simulink library "halin"  (R2021b)
settings: Solver=VariableStepAuto  StartTime=0.0  StopTime=10.0  RelTol=1e-3
undefined symbols (not defined in the file): KHAL_CAN1ABM1E2E_flg, KHAL_CAN1ESC1E2E_flg, KHAL_CAN1ESC5E2E_flg, KHAL_CAN1ESC7E2E_flg, KHAL_CAN1FCM2E2E_flg, KHAL_CAN1FCM3E2E_flg, KHAL_CAN1FCM4E2E_flg, KHAL_CAN3BMS1E2E_flg, KHAL_CAN3BMS6E2E_flg, KHAL_CAN3CCU1E2E_flg, KHAL_CAN3CCU2E2E_flg, KHAL_CAN3MCUF1E2E_flg, KHAL_CAN3MCUR1E2E_flg, KHAL_CAN3Shifter1E2E_flg, TRUE
libraries: simulink x420, FVT_lib x149, hcu_lib x49
(part 9 of 14)

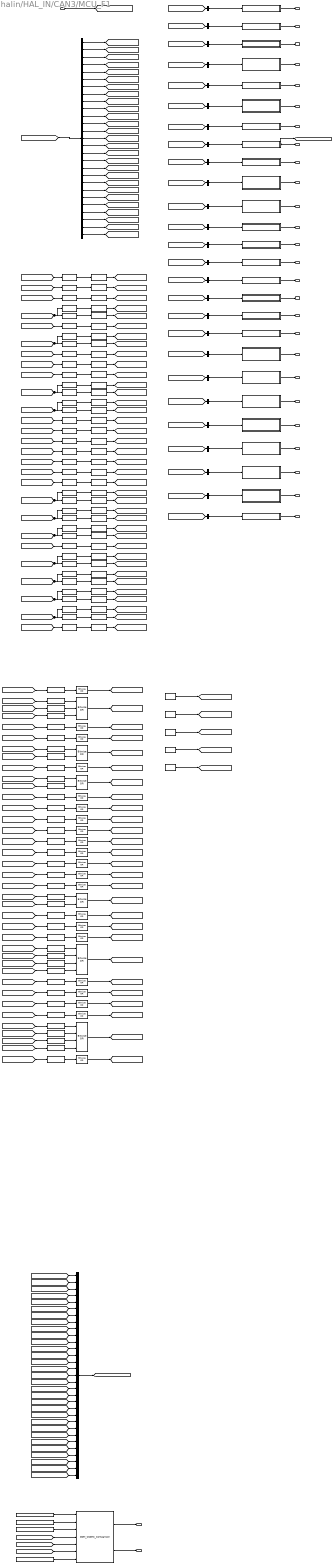
== system halin/HAL_IN/CAN3/MCU_F1 ==
  DT_CAN3_SG_MCU_F1 : Inport
  0x95 : Constant  Value=0x95
  0xf9 : Constant  Value=0xf9
  BitwiseAND{,1..37} (38 alike) : simulink/Logic and Bit Operations/Bitwise Operator  logicop=AND  UseBitMask=on  BitMask=0xFF  BitMaskRealWorld=Stored Integer
  BitwiseOR{,2..3,5,7..15,17..19,21..24,26} (21 alike) : simulink/Logic and Bit Operations/Bitwise Operator  logicop=OR  UseBitMask=off  BitMask=bin2dec('11011001')  BitMaskRealWorld=Stored Integer
  BitwiseOR1 : simulink/Logic and Bit Operations/Bitwise Operator  logicop=OR  UseBitMask=off  NumInputPorts=3  BitMask=bin2dec('11011001')  BitMaskRealWorld=Stored Integer
  BitwiseOR16 : simulink/Logic and Bit Operations/Bitwise Operator  logicop=OR  UseBitMask=off  NumInputPorts=2  BitMask=bin2dec('11011001')  BitMaskRealWorld=Stored Integer
  BitwiseOR20 : simulink/Logic and Bit Operations/Bitwise Operator  logicop=OR  UseBitMask=off  NumInputPorts=4  BitMask=bin2dec('11011001')  BitMaskRealWorld=Stored Integer
  BitwiseOR25 : simulink/Logic and Bit Operations/Bitwise Operator  logicop=OR  UseBitMask=off  NumInputPorts=4  BitMask=bin2dec('11011001')  BitMaskRealWorld=Stored Integer
  BitwiseOR4 : simulink/Logic and Bit Operations/Bitwise Operator  logicop=OR  UseBitMask=off  NumInputPorts=2  BitMask=bin2dec('11011001')  BitMaskRealWorld=Stored Integer
  BitwiseOR6 : simulink/Logic and Bit Operations/Bitwise Operator  logicop=OR  UseBitMask=off  NumInputPorts=2  BitMask=bin2dec('11011001')  BitMaskRealWorld=Stored Integer
  DDM_CS&RC_Comparison : FVT_lib/hal/DDM_CS&RC_Comparison  MsgCycleTime=10
  Data Type Conversion{,1..37} (38 alike) : DataTypeConversion  OutDataTypeStr=uint8
  FrActvDmpDisabSta : Subsystem
  FrEDUDrtSta : Subsystem
  FrEDUOpratingSta : Subsystem
  FrEDURealTMTq : Subsystem
  FrEDURotateDirction : Subsystem
  FrEDUTqReqFbk : Subsystem
  FrMCU1Chksum : Subsystem
  FrMCU1RolCnt : Subsystem
  FrMCUBAT : Subsystem
  FrMCUDCBusCurr : Subsystem
  FrMCUDCBusVolt : Subsystem
  FrMCUDischrgSta : Subsystem
  FrMCUEnaSta : Subsystem
  FrMCUErr : Subsystem
  FrMCUIGNsta : Subsystem
  FrMCUReady : Subsystem
  FrMCUReady4Pre : Subsystem
  FrMCUSysSta : Subsystem
  FrMCUTemp : Subsystem
  FrMotorAvailTq : Subsystem
  FrRegenAvailTq : Subsystem
  FrTMSpd : Subsystem
  FrTMTemp : Subsystem
  FrTMid : Subsystem
  FrTMiq : Subsystem
  KHAL_CAN3MCUF1E2E_flg : Constant  Value=KHAL_CAN3MCUF1E2E_flg
  LeftShift : ArithShift  BitShiftNumber=1  BitShiftDirection=Left
  LeftShift1 : ArithShift  BitShiftNumber=2  BitShiftDirection=Left
  LeftShift{4,6,9..10,12..13,15} (7 alike) : ArithShift  BitShiftDirection=Left
  LeftShift11 : ArithShift  BitShiftNumber=3  BitShiftDirection=Left
  LeftShift14 : ArithShift  BitShiftNumber=1  BitShiftDirection=Left
  LeftShift2 : ArithShift  BitShiftNumber=5  BitShiftDirection=Left
  LeftShift3 : ArithShift  BitShiftNumber=6  BitShiftDirection=Left
  LeftShift5 : ArithShift  BitShiftNumber=4  BitShiftDirection=Left
  LeftShift7 : ArithShift  BitShiftNumber=3  BitShiftDirection=Left
  LeftShift8 : ArithShift  BitShiftNumber=4  BitShiftDirection=Left
  MCUWarnF : Subsystem
  MessageRollingCounter : FVT_lib/hal/MessageRollingCounter  CounterMAX=14  task_time_ms=5  msg_time_ms=10
  Mux : Mux  Inputs=31
  RightShift{,2,4,6,10,14,16,18,20} (9 alike) : ArithShift  BitShiftNumber=8
  RightShift{1,3,5,7,11,15,17,19,21} (9 alike) : ArithShift
  RightShift12 : ArithShift  BitShiftNumber=4
  RightShift13 : ArithShift  BitShiftNumber=-4
  RightShift8 : ArithShift  BitShiftNumber=1
  RightShift9 : ArithShift  BitShiftNumber=-7
  bus_selector : BusSelector  OutputSignals=CAN3_Fr_ActvDmpDisabSta,CAN3_Fr_EDUDrtSta,CAN3_Fr_EDUOpratingSta,CAN3_Fr_EDURealTMTq,CAN3_Fr_EDURotateDirction,CAN3_Fr_EDUTqReqFbk,CAN3_Fr_MCU1Chksum,CAN3_Fr_MCU1RolCnt,CAN3_Fr_MCUBAT,CAN3_Fr_MCUDCBusCurr,CAN3_Fr_MCUDCBusVolt,CAN3_Fr_MCUDischrgSta,CAN3_Fr_MCUEnaSta,CAN3_Fr_MCUErr,CAN3_Fr_MCUIGN_sta,CAN3_Fr_MCUReady,CAN3_Fr_MCUReady4Pre,CAN3_Fr_MCUSysSta,CAN3_Fr_MCUTemp,CAN3_Fr_MotorAvailTq,CAN3_Fr_RegenAvailTq,CAN3_Fr_Reserved_bits,CAN3_Fr_TMSpd,CAN3_Fr_TMTemp,CAN3_Fr_TMid,CAN3_Fr_TMiq,CAN3_MCUWarn_F
  bus_selector1 : BusSelector  OutputSignals=CAN3_Fr_ActvDmpDisabSta
  bus_selector10 : BusSelector  OutputSignals=CAN3_Fr_MCUDCBusCurr
  bus_selector11 : BusSelector  OutputSignals=CAN3_Fr_MCUDCBusVolt
  bus_selector12 : BusSelector  OutputSignals=CAN3_Fr_MCUDischrgSta
  bus_selector13 : BusSelector  OutputSignals=CAN3_Fr_MCUEnaSta
  bus_selector14 : BusSelector  OutputSignals=CAN3_Fr_MCUErr
  bus_selector15 : BusSelector  OutputSignals=CAN3_Fr_MCUIGN_sta
  bus_selector16 : BusSelector  OutputSignals=CAN3_Fr_MCUReady
  bus_selector17 : BusSelector  OutputSignals=CAN3_Fr_MCUReady4Pre
  bus_selector18 : BusSelector  OutputSignals=CAN3_Fr_MCUSysSta
  bus_selector19 : BusSelector  OutputSignals=CAN3_Fr_MCUTemp
  bus_selector2 : BusSelector  OutputSignals=CAN3_Fr_EDUDrtSta
  bus_selector20 : BusSelector  OutputSignals=CAN3_Fr_MotorAvailTq
  bus_selector21 : BusSelector  OutputSignals=CAN3_Fr_RegenAvailTq
  bus_selector22 : BusSelector  OutputSignals=CAN3_Fr_TMSpd
  bus_selector23 : BusSelector  OutputSignals=CAN3_Fr_TMTemp
  bus_selector24 : BusSelector  OutputSignals=CAN3_Fr_TMid
  bus_selector25 : BusSelector  OutputSignals=CAN3_Fr_TMiq
  bus_selector26 : BusSelector  OutputSignals=CAN3_MCUWarn_F
  bus_selector3 : BusSelector  OutputSignals=CAN3_Fr_EDUOpratingSta
  bus_selector4 : BusSelector  OutputSignals=CAN3_Fr_EDURealTMTq
  bus_selector5 : BusSelector  OutputSignals=CAN3_Fr_EDURotateDirction
  bus_selector6 : BusSelector  OutputSignals=CAN3_Fr_EDUTqReqFbk
  bus_selector7 : BusSelector  OutputSignals=CAN3_Fr_MCU1Chksum
  bus_selector8 : BusSelector  OutputSignals=CAN3_Fr_MCU1RolCnt
  bus_selector9 : BusSelector  OutputSignals=CAN3_Fr_MCUBAT
  constant{,1..4} (5 alike) : Constant  Value=0x0  OutDataTypeStr=uint8
  VHAL_MCUF1CSErr_flg : Outport
  VHAL_MCUF1RCErr_flg : Outport  Port=2
  VHAL_FrActvDmpDisabSta_flg : Outport  Port=3
  VHAL_FrEDUDrtSta_flg : Outport  Port=4
  VHAL_FrEDUOpratingSta_flg : Outport  Port=5
  VHAL_FrEDURealTMTq_Nm : Outport  Port=6
  VHAL_FrEDURotateDirction_enum : Outport  Port=7
  VHAL_FrEDUTqReqFbk_Nm : Outport  Port=8
  VHAL_FrMCU1Chksum_enum : Outport  Port=9
  VHAL_FrMCU1RolCnt_enum : Outport  Port=10
  VHAL_FrMCUBAT_V : Outport  Port=11
  VHAL_FrMCUDCBusCurr_A : Outport  Port=12
  VHAL_FrMCUDCBusVolt_V : Outport  Port=13
  VHAL_FrMCUDischrgSta_flg : Outport  Port=14
  VHAL_FrMCUEnaSta_flg : Outport  Port=15
  VHAL_FrMCUErr_enum : Outport  Port=16
  VHAL_FrMCUIGNsta_flg : Outport  Port=17
  VHAL_FrMCUReady_flg : Outport  Port=18
  VHAL_FrMCUReady4Pre_flg : Outport  Port=19
  VHAL_FrMCUSysSta_enum : Outport  Port=20
  VHAL_FrMCUTemp_C : Outport  Port=21
  VHAL_FrMotorAvailTq_Nm : Outport  Port=22
  VHAL_FrRegenAvailTq_Nm : Outport  Port=23
  VHAL_FrTMSpd_rpm : Outport  Port=24
  VHAL_FrTMTemp_C : Outport  Port=25
  VHAL_FrTMid_A : Outport  Port=26
  VHAL_FrTMiq_A : Outport  Port=27
  VHAL_MCUWarnF_enum : Outport  Port=28
  wires:
  DT_CAN3_SG_MCU_F1/1 -> [DT_CAN3_SG_MCU_F1]
  [DT_CAN3_SG_MCU_F1] -> bus_selector/1
  bus_selector/1 -> [CAN3_Fr_ActvDmpDisabSta]  "<CAN3_Fr_ActvDmpDisabSta>"
  [CAN3_Fr_ActvDmpDisabSta] -> LeftShift/1
  LeftShift/1 -> BitwiseAND/1
  BitwiseAND/1 -> [Byte_25_CAN3_Fr_ActvDmpDisabSta]
  bus_selector/2 -> [CAN3_Fr_EDUDrtSta]  "<CAN3_Fr_EDUDrtSta>"
  [CAN3_Fr_EDUDrtSta] -> LeftShift1/1
  LeftShift1/1 -> BitwiseAND1/1
  BitwiseAND1/1 -> [Byte_25_CAN3_Fr_EDUDrtSta]
  bus_selector/3 -> [CAN3_Fr_EDUOpratingSta]  "<CAN3_Fr_EDUOpratingSta>"
  [CAN3_Fr_EDUOpratingSta] -> LeftShift2/1
  LeftShift2/1 -> BitwiseAND2/1
  BitwiseAND2/1 -> [Byte_30_CAN3_Fr_EDUOpratingSta]
  bus_selector/4 -> [CAN3_Fr_EDURealTMTq]  "<CAN3_Fr_EDURealTMTq>"
  [CAN3_Fr_EDURealTMTq] -> RightShift/1, RightShift1/1
  RightShift/1 -> BitwiseAND3/1
  BitwiseAND3/1 -> [Byte_28_CAN3_Fr_EDURealTMTq]
  RightShift1/1 -> BitwiseAND4/1
  BitwiseAND4/1 -> [Byte_29_CAN3_Fr_EDURealTMTq]
  bus_selector/5 -> [CAN3_Fr_EDURotateDirction]  "<CAN3_Fr_EDURotateDirction>"
  [CAN3_Fr_EDURotateDirction] -> LeftShift3/1
  LeftShift3/1 -> BitwiseAND5/1
  BitwiseAND5/1 -> [Byte_30_CAN3_Fr_EDURotateDirction]
  bus_selector/6 -> [CAN3_Fr_EDUTqReqFbk]  "<CAN3_Fr_EDUTqReqFbk>"
  [CAN3_Fr_EDUTqReqFbk] -> RightShift2/1, RightShift3/1
  RightShift2/1 -> BitwiseAND6/1
  BitwiseAND6/1 -> [Byte_30_CAN3_Fr_EDUTqReqFbk]
  RightShift3/1 -> BitwiseAND7/1
  BitwiseAND7/1 -> [Byte_31_CAN3_Fr_EDUTqReqFbk]
  bus_selector/7 -> [CAN3_Fr_MCU1Chksum]  "<CAN3_Fr_MCU1Chksum>"
  [CAN3_Fr_MCU1Chksum] -> LeftShift4/1
  LeftShift4/1 -> BitwiseAND8/1
  BitwiseAND8/1 -> [Byte_0_CAN3_Fr_MCU1Chksum]
  bus_selector/8 -> [CAN3_Fr_MCU1RolCnt]  "<CAN3_Fr_MCU1RolCnt>"
  [CAN3_Fr_MCU1RolCnt] -> LeftShift5/1
  LeftShift5/1 -> BitwiseAND9/1
  BitwiseAND9/1 -> [Byte_1_CAN3_Fr_MCU1RolCnt]
  bus_selector/9 -> [CAN3_Fr_MCUBAT]  "<CAN3_Fr_MCUBAT>"
  [CAN3_Fr_MCUBAT] -> LeftShift6/1
  LeftShift6/1 -> BitwiseAND10/1
  BitwiseAND10/1 -> [Byte_8_CAN3_Fr_MCUBAT]
  bus_selector/10 -> [CAN3_Fr_MCUDCBusCurr]  "<CAN3_Fr_MCUDCBusCurr>"
  [CAN3_Fr_MCUDCBusCurr] -> RightShift4/1, RightShift5/1
  RightShift4/1 -> BitwiseAND11/1
  BitwiseAND11/1 -> [Byte_21_CAN3_Fr_MCUDCBusCurr]
  RightShift5/1 -> BitwiseAND12/1
  BitwiseAND12/1 -> [Byte_22_CAN3_Fr_MCUDCBusCurr]
  bus_selector/11 -> [CAN3_Fr_MCUDCBusVolt]  "<CAN3_Fr_MCUDCBusVolt>"
  [CAN3_Fr_MCUDCBusVolt] -> RightShift6/1, RightShift7/1
  RightShift6/1 -> BitwiseAND13/1
  BitwiseAND13/1 -> [Byte_23_CAN3_Fr_MCUDCBusVolt]
  RightShift7/1 -> BitwiseAND14/1
  BitwiseAND14/1 -> [Byte_24_CAN3_Fr_MCUDCBusVolt]
  bus_selector/12 -> [CAN3_Fr_MCUDischrgSta]  "<CAN3_Fr_MCUDischrgSta>"
  [CAN3_Fr_MCUDischrgSta] -> LeftShift7/1
  LeftShift7/1 -> BitwiseAND15/1
  BitwiseAND15/1 -> [Byte_25_CAN3_Fr_MCUDischrgSta]
  bus_selector/13 -> [CAN3_Fr_MCUEnaSta]  "<CAN3_Fr_MCUEnaSta>"
  [CAN3_Fr_MCUEnaSta] -> LeftShift8/1
  LeftShift8/1 -> BitwiseAND16/1
  BitwiseAND16/1 -> [Byte_30_CAN3_Fr_MCUEnaSta]
  bus_selector/14 -> [CAN3_Fr_MCUErr]  "<CAN3_Fr_MCUErr>"
  [CAN3_Fr_MCUErr] -> LeftShift9/1
  LeftShift9/1 -> BitwiseAND17/1
  BitwiseAND17/1 -> [Byte_17_CAN3_Fr_MCUErr]
  bus_selector/15 -> [CAN3_Fr_MCUIGN_sta]  "<CAN3_Fr_MCUIGN_sta>"
  [CAN3_Fr_MCUIGN_sta] -> LeftShift10/1
  LeftShift10/1 -> BitwiseAND18/1
  BitwiseAND18/1 -> [Byte_9_CAN3_Fr_MCUIGN_sta]
  bus_selector/16 -> [CAN3_Fr_MCUReady]  "<CAN3_Fr_MCUReady>"
  [CAN3_Fr_MCUReady] -> LeftShift11/1
  LeftShift11/1 -> BitwiseAND19/1
  BitwiseAND19/1 -> [Byte_1_CAN3_Fr_MCUReady]
  bus_selector/17 -> [CAN3_Fr_MCUReady4Pre]  "<CAN3_Fr_MCUReady4Pre>"
  [CAN3_Fr_MCUReady4Pre] -> LeftShift12/1
  LeftShift12/1 -> BitwiseAND20/1
  BitwiseAND20/1 -> [Byte_25_CAN3_Fr_MCUReady4Pre]
  bus_selector/18 -> [CAN3_Fr_MCUSysSta]  "<CAN3_Fr_MCUSysSta>"
  [CAN3_Fr_MCUSysSta] -> LeftShift13/1
  LeftShift13/1 -> BitwiseAND21/1
  BitwiseAND21/1 -> [Byte_7_CAN3_Fr_MCUSysSta]
  bus_selector/19 -> [CAN3_Fr_MCUTemp]  "<CAN3_Fr_MCUTemp>"
  [CAN3_Fr_MCUTemp] -> RightShift8/1, RightShift9/1
  RightShift8/1 -> BitwiseAND22/1
  BitwiseAND22/1 -> [Byte_20_CAN3_Fr_MCUTemp]
  RightShift9/1 -> BitwiseAND23/1
  BitwiseAND23/1 -> [Byte_21_CAN3_Fr_MCUTemp]
  bus_selector/20 -> [CAN3_Fr_MotorAvailTq]  "<CAN3_Fr_MotorAvailTq>"
  [CAN3_Fr_MotorAvailTq] -> RightShift10/1, RightShift11/1
  RightShift10/1 -> BitwiseAND24/1
  BitwiseAND24/1 -> [Byte_11_CAN3_Fr_MotorAvailTq]
  RightShift11/1 -> BitwiseAND25/1
  BitwiseAND25/1 -> [Byte_12_CAN3_Fr_MotorAvailTq]
  bus_selector/21 -> [CAN3_Fr_RegenAvailTq]  "<CAN3_Fr_RegenAvailTq>"
  [CAN3_Fr_RegenAvailTq] -> RightShift12/1, RightShift13/1
  RightShift12/1 -> BitwiseAND26/1
  BitwiseAND26/1 -> [Byte_10_CAN3_Fr_RegenAvailTq]
  RightShift13/1 -> BitwiseAND27/1
  BitwiseAND27/1 -> [Byte_11_CAN3_Fr_RegenAvailTq]
  bus_selector/22 -> [CAN3_Fr_Reserved_bits]  "<CAN3_Fr_Reserved_bits>"
  [CAN3_Fr_Reserved_bits] -> LeftShift14/1
  LeftShift14/1 -> BitwiseAND28/1
  BitwiseAND28/1 -> [Byte_9_CAN3_Fr_Reserved_bits]
  bus_selector/23 -> [CAN3_Fr_TMSpd]  "<CAN3_Fr_TMSpd>"
  [CAN3_Fr_TMSpd] -> RightShift14/1, RightShift15/1
  RightShift14/1 -> BitwiseAND29/1
  BitwiseAND29/1 -> [Byte_26_CAN3_Fr_TMSpd]
  RightShift15/1 -> BitwiseAND30/1
  BitwiseAND30/1 -> [Byte_27_CAN3_Fr_TMSpd]
  bus_selector/24 -> [CAN3_Fr_TMTemp]  "<CAN3_Fr_TMTemp>"
  [CAN3_Fr_TMTemp] -> RightShift16/1, RightShift17/1
  RightShift16/1 -> BitwiseAND31/1
  BitwiseAND31/1 -> [Byte_18_CAN3_Fr_TMTemp]
  RightShift17/1 -> BitwiseAND32/1
  BitwiseAND32/1 -> [Byte_19_CAN3_Fr_TMTemp]
  bus_selector/25 -> [CAN3_Fr_TMid]  "<CAN3_Fr_TMid>"
  [CAN3_Fr_TMid] -> RightShift18/1, RightShift19/1
  RightShift18/1 -> BitwiseAND33/1
  BitwiseAND33/1 -> [Byte_15_CAN3_Fr_TMid]
  RightShift19/1 -> BitwiseAND34/1
  BitwiseAND34/1 -> [Byte_16_CAN3_Fr_TMid]
  bus_selector/26 -> [CAN3_Fr_TMiq]  "<CAN3_Fr_TMiq>"
  [CAN3_Fr_TMiq] -> RightShift20/1, RightShift21/1
  RightShift20/1 -> BitwiseAND35/1
  BitwiseAND35/1 -> [Byte_13_CAN3_Fr_TMiq]
  RightShift21/1 -> BitwiseAND36/1
  BitwiseAND36/1 -> [Byte_14_CAN3_Fr_TMiq]
  bus_selector/27 -> [CAN3_MCUWarn_F]  "<CAN3_MCUWarn_F>"
  [CAN3_MCUWarn_F] -> LeftShift15/1
  LeftShift15/1 -> BitwiseAND37/1
  BitwiseAND37/1 -> [Byte_1_CAN3_MCUWarn_F]
  Data Type Conversion/1 -> BitwiseOR/1
  [Byte_0_CAN3_Fr_MCU1Chksum] -> Data Type Conversion/1
  BitwiseOR/1 -> [Byte_0]
  Data Type Conversion1/1 -> BitwiseOR1/1
  [Byte_1_CAN3_Fr_MCU1RolCnt] -> Data Type Conversion1/1
  Data Type Conversion2/1 -> BitwiseOR1/2
  [Byte_1_CAN3_Fr_MCUReady] -> Data Type Conversion2/1
  Data Type Conversion3/1 -> BitwiseOR1/3
  [Byte_1_CAN3_MCUWarn_F] -> Data Type Conversion3/1
  BitwiseOR1/1 -> [Byte_1]
  constant/1 -> [Byte_2]
  constant1/1 -> [Byte_3]
  constant2/1 -> [Byte_4]
  constant3/1 -> [Byte_5]
  constant4/1 -> [Byte_6]
  Data Type Conversion4/1 -> BitwiseOR2/1
  [Byte_7_CAN3_Fr_MCUSysSta] -> Data Type Conversion4/1
  BitwiseOR2/1 -> [Byte_7]
  Data Type Conversion5/1 -> BitwiseOR3/1
  [Byte_8_CAN3_Fr_MCUBAT] -> Data Type Conversion5/1
  BitwiseOR3/1 -> [Byte_8]
  Data Type Conversion6/1 -> BitwiseOR4/1
  [Byte_9_CAN3_Fr_MCUIGN_sta] -> Data Type Conversion6/1
  Data Type Conversion7/1 -> BitwiseOR4/2
  [Byte_9_CAN3_Fr_Reserved_bits] -> Data Type Conversion7/1
  BitwiseOR4/1 -> [Byte_9]
  Data Type Conversion8/1 -> BitwiseOR5/1
  [Byte_10_CAN3_Fr_RegenAvailTq] -> Data Type Conversion8/1
  BitwiseOR5/1 -> [Byte_10]
  Data Type Conversion9/1 -> BitwiseOR6/1
  [Byte_11_CAN3_Fr_MotorAvailTq] -> Data Type Conversion9/1
  Data Type Conversion10/1 -> BitwiseOR6/2
  [Byte_11_CAN3_Fr_RegenAvailTq] -> Data Type Conversion10/1
  BitwiseOR6/1 -> [Byte_11]
  Data Type Conversion11/1 -> BitwiseOR7/1
  [Byte_12_CAN3_Fr_MotorAvailTq] -> Data Type Conversion11/1
  BitwiseOR7/1 -> [Byte_12]
  Data Type Conversion12/1 -> BitwiseOR8/1
  [Byte_13_CAN3_Fr_TMiq] -> Data Type Conversion12/1
  BitwiseOR8/1 -> [Byte_13]
  Data Type Conversion13/1 -> BitwiseOR9/1
  [Byte_14_CAN3_Fr_TMiq] -> Data Type Conversion13/1
  BitwiseOR9/1 -> [Byte_14]
  Data Type Conversion14/1 -> BitwiseOR10/1
  [Byte_15_CAN3_Fr_TMid] -> Data Type Conversion14/1
  BitwiseOR10/1 -> [Byte_15]
  Data Type Conversion15/1 -> BitwiseOR11/1
  [Byte_16_CAN3_Fr_TMid] -> Data Type Conversion15/1
  BitwiseOR11/1 -> [Byte_16]
  Data Type Conversion16/1 -> BitwiseOR12/1
  [Byte_17_CAN3_Fr_MCUErr] -> Data Type Conversion16/1
  BitwiseOR12/1 -> [Byte_17]
  Data Type Conversion17/1 -> BitwiseOR13/1
  [Byte_18_CAN3_Fr_TMTemp] -> Data Type Conversion17/1
  BitwiseOR13/1 -> [Byte_18]
  Data Type Conversion18/1 -> BitwiseOR14/1
  [Byte_19_CAN3_Fr_TMTemp] -> Data Type Conversion18/1
  BitwiseOR14/1 -> [Byte_19]
  Data Type Conversion19/1 -> BitwiseOR15/1
  [Byte_20_CAN3_Fr_MCUTemp] -> Data Type Conversion19/1
  BitwiseOR15/1 -> [Byte_20]
  Data Type Conversion20/1 -> BitwiseOR16/1
  [Byte_21_CAN3_Fr_MCUDCBusCurr] -> Data Type Conversion20/1
  Data Type Conversion21/1 -> BitwiseOR16/2
  [Byte_21_CAN3_Fr_MCUTemp] -> Data Type Conversion21/1
  BitwiseOR16/1 -> [Byte_21]
  Data Type Conversion22/1 -> BitwiseOR17/1
  [Byte_22_CAN3_Fr_MCUDCBusCurr] -> Data Type Conversion22/1
  BitwiseOR17/1 -> [Byte_22]
  Data Type Conversion23/1 -> BitwiseOR18/1
  [Byte_23_CAN3_Fr_MCUDCBusVolt] -> Data Type Conversion23/1
  BitwiseOR18/1 -> [Byte_23]
  Data Type Conversion24/1 -> BitwiseOR19/1
  [Byte_24_CAN3_Fr_MCUDCBusVolt] -> Data Type Conversion24/1
  BitwiseOR19/1 -> [Byte_24]
  Data Type Conversion25/1 -> BitwiseOR20/1
  [Byte_25_CAN3_Fr_ActvDmpDisabSta] -> Data Type Conversion25/1
  Data Type Conversion26/1 -> BitwiseOR20/2
  [Byte_25_CAN3_Fr_EDUDrtSta] -> Data Type Conversion26/1
  Data Type Conversion27/1 -> BitwiseOR20/3
  [Byte_25_CAN3_Fr_MCUDischrgSta] -> Data Type Conversion27/1
  Data Type Conversion28/1 -> BitwiseOR20/4
  [Byte_25_CAN3_Fr_MCUReady4Pre] -> Data Type Conversion28/1
  BitwiseOR20/1 -> [Byte_25]
  Data Type Conversion29/1 -> BitwiseOR21/1
  [Byte_26_CAN3_Fr_TMSpd] -> Data Type Conversion29/1
  BitwiseOR21/1 -> [Byte_26]
  Data Type Conversion30/1 -> BitwiseOR22/1
  [Byte_27_CAN3_Fr_TMSpd] -> Data Type Conversion30/1
  BitwiseOR22/1 -> [Byte_27]
  Data Type Conversion31/1 -> BitwiseOR23/1
  [Byte_28_CAN3_Fr_EDURealTMTq] -> Data Type Conversion31/1
  BitwiseOR23/1 -> [Byte_28]
  Data Type Conversion32/1 -> BitwiseOR24/1
  [Byte_29_CAN3_Fr_EDURealTMTq] -> Data Type Conversion32/1
  BitwiseOR24/1 -> [Byte_29]
  Data Type Conversion33/1 -> BitwiseOR25/1
  [Byte_30_CAN3_Fr_EDUOpratingSta] -> Data Type Conversion33/1
  Data Type Conversion34/1 -> BitwiseOR25/2
  [Byte_30_CAN3_Fr_EDURotateDirction] -> Data Type Conversion34/1
  Data Type Conversion35/1 -> BitwiseOR25/3
  [Byte_30_CAN3_Fr_EDUTqReqFbk] -> Data Type Conversion35/1
  Data Type Conversion36/1 -> BitwiseOR25/4
  [Byte_30_CAN3_Fr_MCUEnaSta] -> Data Type Conversion36/1
  BitwiseOR25/1 -> [Byte_30]
  Data Type Conversion37/1 -> BitwiseOR26/1
  [Byte_31_CAN3_Fr_EDUTqReqFbk] -> Data Type Conversion37/1
  BitwiseOR26/1 -> [Byte_31]
  [Byte_1] -> Mux/1
  [Byte_2] -> Mux/2
  [Byte_3] -> Mux/3
  [Byte_4] -> Mux/4
  [Byte_5] -> Mux/5
  [Byte_6] -> Mux/6
  [Byte_7] -> Mux/7
  [Byte_8] -> Mux/8
  [Byte_9] -> Mux/9
  [Byte_10] -> Mux/10
  [Byte_11] -> Mux/11
  [Byte_12] -> Mux/12
  [Byte_13] -> Mux/13
  [Byte_14] -> Mux/14
  [Byte_15] -> Mux/15
  [Byte_16] -> Mux/16
  [Byte_17] -> Mux/17
  [Byte_18] -> Mux/18
  [Byte_19] -> Mux/19
  [Byte_20] -> Mux/20
  [Byte_21] -> Mux/21
  [Byte_22] -> Mux/22
  [Byte_23] -> Mux/23
  [Byte_24] -> Mux/24
  [Byte_25] -> Mux/25
  [Byte_26] -> Mux/26
  [Byte_27] -> Mux/27
  [Byte_28] -> Mux/28
  [Byte_29] -> Mux/29
  [Byte_30] -> Mux/30
  [Byte_31] -> Mux/31
  Mux/1 -> [VHAL_CAN3MCUF1noCS_raw]
  KHAL_CAN3MCUF1E2E_flg/1 -> DDM_CS&RC_Comparison/1
  0xf9/1 -> DDM_CS&RC_Comparison/2
  0x95/1 -> DDM_CS&RC_Comparison/3
  [VHAL_CAN3MCUF1noCS_raw] -> DDM_CS&RC_Comparison/4
  [Byte_0] -> DDM_CS&RC_Comparison/5
  [RC_ECU] -> DDM_CS&RC_Comparison/6
  MessageRollingCounter/1 -> DDM_CS&RC_Comparison/7
  DDM_CS&RC_Comparison/1 -> VHAL_MCUF1CSErr_flg/1
  DDM_CS&RC_Comparison/2 -> VHAL_MCUF1RCErr_flg/1
  [DT_CAN3_SG_MCU_F1] -> bus_selector1/1
  bus_selector1/1 -> FrActvDmpDisabSta/1(Fr_ActvDmpDisabSta)  "<CAN3_Fr_ActvDmpDisabSta>"
  FrActvDmpDisabSta/1(VHAL_FrActvDmpDisabSta_flg) -> VHAL_FrActvDmpDisabSta_flg/1
  [DT_CAN3_SG_MCU_F1] -> bus_selector2/1
  bus_selector2/1 -> FrEDUDrtSta/1(Fr_EDUDrtSta)  "<CAN3_Fr_EDUDrtSta>"
  FrEDUDrtSta/1(VHAL_FrEDUDrtSta_flg) -> VHAL_FrEDUDrtSta_flg/1
  [DT_CAN3_SG_MCU_F1] -> bus_selector3/1
  bus_selector3/1 -> FrEDUOpratingSta/1(Fr_EDUOpratingSta)  "<CAN3_Fr_EDUOpratingSta>"
  FrEDUOpratingSta/1(VHAL_FrEDUOpratingSta_flg) -> VHAL_FrEDUOpratingSta_flg/1
  [DT_CAN3_SG_MCU_F1] -> bus_selector4/1
  bus_selector4/1 -> FrEDURealTMTq/1(Fr_EDURealTMTq)  "<CAN3_Fr_EDURealTMTq>"
  FrEDURealTMTq/1(VHAL_FrEDURealTMTq_Nm) -> VHAL_FrEDURealTMTq_Nm/1
  [DT_CAN3_SG_MCU_F1] -> bus_selector5/1
  bus_selector5/1 -> FrEDURotateDirction/1(Fr_EDURotateDirction)  "<CAN3_Fr_EDURotateDirction>"
  FrEDURotateDirction/1(VHAL_FrEDURotateDirction_enum) -> VHAL_FrEDURotateDirction_enum/1
  [DT_CAN3_SG_MCU_F1] -> bus_selector6/1
  bus_selector6/1 -> FrEDUTqReqFbk/1(Fr_EDUTqReqFbk)  "<CAN3_Fr_EDUTqReqFbk>"
  FrEDUTqReqFbk/1(VHAL_FrEDUTqReqFbk_Nm) -> VHAL_FrEDUTqReqFbk_Nm/1
  [DT_CAN3_SG_MCU_F1] -> bus_selector7/1
  bus_selector7/1 -> FrMCU1Chksum/1(Fr_MCU1Chksum)  "<CAN3_Fr_MCU1Chksum>"
  FrMCU1Chksum/1(VHAL_FrMCU1Chksum_enum) -> VHAL_FrMCU1Chksum_enum/1
  [DT_CAN3_SG_MCU_F1] -> bus_selector8/1
  bus_selector8/1 -> FrMCU1RolCnt/1(Fr_MCU1RolCnt)  "<CAN3_Fr_MCU1RolCnt>"
  FrMCU1RolCnt/1(VHAL_FrMCU1RolCnt_enum) -> VHAL_FrMCU1RolCnt_enum/1, [RC_ECU]
  [DT_CAN3_SG_MCU_F1] -> bus_selector9/1
  bus_selector9/1 -> FrMCUBAT/1(Fr_MCUBAT)  "<CAN3_Fr_MCUBAT>"
  FrMCUBAT/1(VHAL_FrMCUBAT_V) -> VHAL_FrMCUBAT_V/1
  [DT_CAN3_SG_MCU_F1] -> bus_selector10/1
  bus_selector10/1 -> FrMCUDCBusCurr/1(Fr_MCUDCBusCurr)  "<CAN3_Fr_MCUDCBusCurr>"
  FrMCUDCBusCurr/1(VHAL_FrMCUDCBusCurr_A) -> VHAL_FrMCUDCBusCurr_A/1
  [DT_CAN3_SG_MCU_F1] -> bus_selector11/1
  bus_selector11/1 -> FrMCUDCBusVolt/1(Fr_MCUDCBusVolt)  "<CAN3_Fr_MCUDCBusVolt>"
  FrMCUDCBusVolt/1(VHAL_FrMCUDCBusVolt_V) -> VHAL_FrMCUDCBusVolt_V/1
  [DT_CAN3_SG_MCU_F1] -> bus_selector12/1
  bus_selector12/1 -> FrMCUDischrgSta/1(Fr_MCUDischrgSta)  "<CAN3_Fr_MCUDischrgSta>"
  FrMCUDischrgSta/1(VHAL_FrMCUDischrgSta_flg) -> VHAL_FrMCUDischrgSta_flg/1
  [DT_CAN3_SG_MCU_F1] -> bus_selector13/1
  bus_selector13/1 -> FrMCUEnaSta/1(Fr_MCUEnaSta)  "<CAN3_Fr_MCUEnaSta>"
  FrMCUEnaSta/1(VHAL_FrMCUEnaSta_flg) -> VHAL_FrMCUEnaSta_flg/1
  [DT_CAN3_SG_MCU_F1] -> bus_selector14/1
  bus_selector14/1 -> FrMCUErr/1(Fr_MCUErr)  "<CAN3_Fr_MCUErr>"
  FrMCUErr/1(VHAL_FrMCUErr_enum) -> VHAL_FrMCUErr_enum/1
  [DT_CAN3_SG_MCU_F1] -> bus_selector15/1
  bus_selector15/1 -> FrMCUIGNsta/1(Fr_MCUIGN_sta)  "<CAN3_Fr_MCUIGN_sta>"
  FrMCUIGNsta/1(VHAL_FrMCUIGNsta_flg) -> VHAL_FrMCUIGNsta_flg/1
  [DT_CAN3_SG_MCU_F1] -> bus_selector16/1
  bus_selector16/1 -> FrMCUReady/1(Fr_MCUReady)  "<CAN3_Fr_MCUReady>"
  FrMCUReady/1(VHAL_FrMCUReady_flg) -> VHAL_FrMCUReady_flg/1
  [DT_CAN3_SG_MCU_F1] -> bus_selector17/1
  bus_selector17/1 -> FrMCUReady4Pre/1(Fr_MCUReady4Pre)  "<CAN3_Fr_MCUReady4Pre>"
  FrMCUReady4Pre/1(VHAL_FrMCUReady4Pre_flg) -> VHAL_FrMCUReady4Pre_flg/1
  [DT_CAN3_SG_MCU_F1] -> bus_selector18/1
  bus_selector18/1 -> FrMCUSysSta/1(Fr_MCUSysSta)  "<CAN3_Fr_MCUSysSta>"
  FrMCUSysSta/1(VHAL_FrMCUSysSta_enum) -> VHAL_FrMCUSysSta_enum/1
  [DT_CAN3_SG_MCU_F1] -> bus_selector19/1
  bus_selector19/1 -> FrMCUTemp/1(Fr_MCUTemp)  "<CAN3_Fr_MCUTemp>"
  FrMCUTemp/1(VHAL_FrMCUTemp_C) -> VHAL_FrMCUTemp_C/1
  [DT_CAN3_SG_MCU_F1] -> bus_selector20/1
  bus_selector20/1 -> FrMotorAvailTq/1(Fr_MotorAvailTq)  "<CAN3_Fr_MotorAvailTq>"
  FrMotorAvailTq/1(VHAL_FrMotorAvailTq_Nm) -> VHAL_FrMotorAvailTq_Nm/1
  [DT_CAN3_SG_MCU_F1] -> bus_selector21/1
  bus_selector21/1 -> FrRegenAvailTq/1(Fr_RegenAvailTq)  "<CAN3_Fr_RegenAvailTq>"
  FrRegenAvailTq/1(VHAL_FrRegenAvailTq_Nm) -> VHAL_FrRegenAvailTq_Nm/1
  [DT_CAN3_SG_MCU_F1] -> bus_selector22/1
  bus_selector22/1 -> FrTMSpd/1(Fr_TMSpd)  "<CAN3_Fr_TMSpd>"
  FrTMSpd/1(VHAL_FrTMSpd_rpm) -> VHAL_FrTMSpd_rpm/1
  [DT_CAN3_SG_MCU_F1] -> bus_selector23/1
  bus_selector23/1 -> FrTMTemp/1(Fr_TMTemp)  "<CAN3_Fr_TMTemp>"
  FrTMTemp/1(VHAL_FrTMTemp_C) -> VHAL_FrTMTemp_C/1
  [DT_CAN3_SG_MCU_F1] -> bus_selector24/1
  bus_selector24/1 -> FrTMid/1(Fr_TMid)  "<CAN3_Fr_TMid>"
  FrTMid/1(VHAL_FrTMid_A) -> VHAL_FrTMid_A/1
  [DT_CAN3_SG_MCU_F1] -> bus_selector25/1
  bus_selector25/1 -> FrTMiq/1(Fr_TMiq)  "<CAN3_Fr_TMiq>"
  FrTMiq/1(VHAL_FrTMiq_A) -> VHAL_FrTMiq_A/1
  [DT_CAN3_SG_MCU_F1] -> bus_selector26/1
  bus_selector26/1 -> MCUWarnF/1(MCUWarn_F)  "<CAN3_MCUWarn_F>"
  MCUWarnF/1(VHAL_MCUWarnF_enum) -> VHAL_MCUWarnF_enum/1

== system halin/HAL_IN/CAN3/MCU_F2 ==
  DT_CAN3_SG_MCU_F2 : Inport
  FrCoolanttempReq : Subsystem
  FrEOPSpdSet : Subsystem
  FrFailcode1 : Subsystem
  FrFailcode2 : Subsystem
  FrFailcodehistory1 : Subsystem
  FrFailcodehistory2 : Subsystem
  FrLLCTemp : Subsystem
  FrLLCflowReq : Subsystem
  FrMCUTempWarn : Subsystem
  FrTMTempWarn : Subsystem
  bus_selector : BusSelector  OutputSignals=CAN3_Fr_CoolanttempReq
  bus_selector1 : BusSelector  OutputSignals=CAN3_Fr_EOP_SpdSet
  bus_selector2 : BusSelector  OutputSignals=CAN3_Fr_Failcode1
  bus_selector3 : BusSelector  OutputSignals=CAN3_Fr_Failcode2
  bus_selector4 : BusSelector  OutputSignals=CAN3_Fr_Failcodehistory1
  bus_selector5 : BusSelector  OutputSignals=CAN3_Fr_Failcodehistory2
  bus_selector6 : BusSelector  OutputSignals=CAN3_Fr_LLCTemp
  bus_selector7 : BusSelector  OutputSignals=CAN3_Fr_LLCflowReq
  bus_selector8 : BusSelector  OutputSignals=CAN3_Fr_MCUTempWarn
  bus_selector9 : BusSelector  OutputSignals=CAN3_Fr_TMTempWarn
  VHAL_FrCoolanttempReq_C : Outport
  VHAL_FrEOPSpdSet_rpm : Outport  Port=2
  VHAL_FrFailcode1_enum : Outport  Port=3
  VHAL_FrFailcode2_enum : Outport  Port=4
  VHAL_FrFailcodehistory1_enum : Outport  Port=5
  VHAL_FrFailcodehistory2_enum : Outport  Port=6
  VHAL_FrLLCTemp_C : Outport  Port=7
  VHAL_FrLLCflowReq_Lpmin : Outport  Port=8
  VHAL_FrMCUTempWarn_enum : Outport  Port=9
  VHAL_FrTMTempWarn_enum : Outport  Port=10
  wires:
  DT_CAN3_SG_MCU_F2/1 -> [DT_CAN3_SG_MCU_F2]
  [DT_CAN3_SG_MCU_F2] -> bus_selector/1
  bus_selector/1 -> FrCoolanttempReq/1(Fr_CoolanttempReq)  "<CAN3_Fr_CoolanttempReq>"
  FrCoolanttempReq/1(VHAL_FrCoolanttempReq_C) -> VHAL_FrCoolanttempReq_C/1
  [DT_CAN3_SG_MCU_F2] -> bus_selector1/1
  bus_selector1/1 -> FrEOPSpdSet/1(Fr_EOP_SpdSet)  "<CAN3_Fr_EOP_SpdSet>"
  FrEOPSpdSet/1(VHAL_FrEOPSpdSet_rpm) -> VHAL_FrEOPSpdSet_rpm/1
  [DT_CAN3_SG_MCU_F2] -> bus_selector2/1
  bus_selector2/1 -> FrFailcode1/1(Fr_Failcode1)  "<CAN3_Fr_Failcode1>"
  FrFailcode1/1(VHAL_FrFailcode1_enum) -> VHAL_FrFailcode1_enum/1
  [DT_CAN3_SG_MCU_F2] -> bus_selector3/1
  bus_selector3/1 -> FrFailcode2/1(Fr_Failcode2)  "<CAN3_Fr_Failcode2>"
  FrFailcode2/1(VHAL_FrFailcode2_enum) -> VHAL_FrFailcode2_enum/1
  [DT_CAN3_SG_MCU_F2] -> bus_selector4/1
  bus_selector4/1 -> FrFailcodehistory1/1(Fr_Failcodehistory1)  "<CAN3_Fr_Failcodehistory1>"
  FrFailcodehistory1/1(VHAL_FrFailcodehistory1_enum) -> VHAL_FrFailcodehistory1_enum/1
  [DT_CAN3_SG_MCU_F2] -> bus_selector5/1
  bus_selector5/1 -> FrFailcodehistory2/1(Fr_Failcodehistory2)  "<CAN3_Fr_Failcodehistory2>"
  FrFailcodehistory2/1(VHAL_FrFailcodehistory2_enum) -> VHAL_FrFailcodehistory2_enum/1
  [DT_CAN3_SG_MCU_F2] -> bus_selector6/1
  bus_selector6/1 -> FrLLCTemp/1(Fr_LLCTemp)  "<CAN3_Fr_LLCTemp>"
  FrLLCTemp/1(VHAL_FrLLCTemp_C) -> VHAL_FrLLCTemp_C/1
  [DT_CAN3_SG_MCU_F2] -> bus_selector7/1
  bus_selector7/1 -> FrLLCflowReq/1(Fr_LLCflowReq)  "<CAN3_Fr_LLCflowReq>"
  FrLLCflowReq/1(VHAL_FrLLCflowReq_Lpmin) -> VHAL_FrLLCflowReq_Lpmin/1
  [DT_CAN3_SG_MCU_F2] -> bus_selector8/1
  bus_selector8/1 -> FrMCUTempWarn/1(Fr_MCUTempWarn)  "<CAN3_Fr_MCUTempWarn>"
  FrMCUTempWarn/1(VHAL_FrMCUTempWarn_enum) -> VHAL_FrMCUTempWarn_enum/1
  [DT_CAN3_SG_MCU_F2] -> bus_selector9/1
  bus_selector9/1 -> FrTMTempWarn/1(Fr_TMTempWarn)  "<CAN3_Fr_TMTempWarn>"
  FrTMTempWarn/1(VHAL_FrTMTempWarn_enum) -> VHAL_FrTMTempWarn_enum/1
